simulink model "ex2_5"  (R2022a)
settings: Solver=VariableStepAuto  StartTime=0.0  StopTime=800  RelTol=1e-3
settings Model: Creator=Xinrui  LastModifiedBy=Xinrui

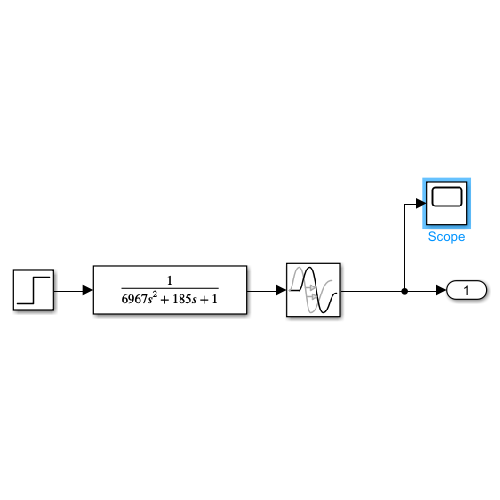
[thumbnail: Simulink's stored preview of the top-level diagram]
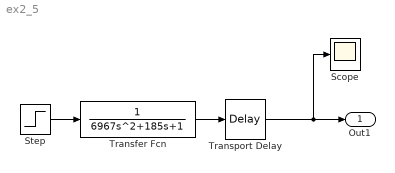
== system ex2_5 ==
  Scope : Scope
  Step : Step  Time=0  After=20  SampleTime=0
  Transfer Fcn : TransferFcn  Denominator=[6967 185 1]
  Transport Delay : TransportDelay  DelayTime=10
  Out1 : Outport
  wires:
  Step/1 -> Transfer Fcn/1
  Transfer Fcn/1 -> Transport Delay/1
  Transport Delay/1 -> Scope/1, Out1/1
